simulink model "Q5_MSD"  (R2024b)
settings: Solver=VariableStepAuto  StartTime=0.0  StopTime=10.0  RelTol=1e-3
settings Model: Creator=chall  LastModifiedBy=chall
settings RTWCC: GPUComputeCapability=3.5

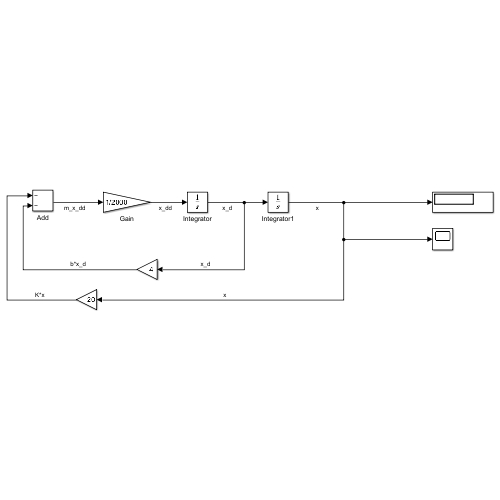
[thumbnail: Simulink's stored preview of the top-level diagram]
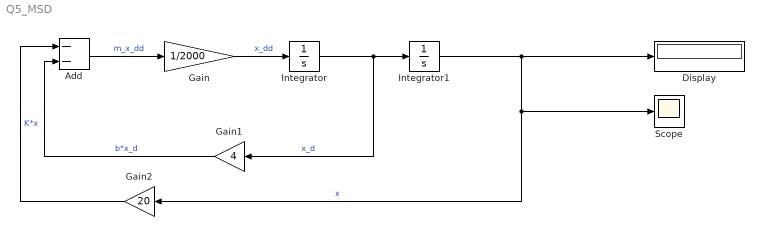
== system Q5_MSD ==
  Add : Sum  Inputs=--
  Display : Display
  Gain : Gain  Gain=1/2000
  Gain1 : Gain  Gain=4
  Gain2 : Gain  Gain=20
  Integrator : Integrator
  Integrator1 : Integrator  InitialCondition=0.1
  Scope : Scope
  wires:
  Add/1 -> Gain/1  "m_x_dd"
  Gain/1 -> Integrator/1  "x_dd"
  Integrator/1 -> Gain1/1, Integrator1/1  "x_d"
  Integrator1/1 -> Scope/1, Gain2/1, Display/1  "x"
  Gain1/1 -> Add/2  "b*x_d"
  Gain2/1 -> Add/1  "K*x"
